simulink model "Constant_TestGen45"  (R2017b)
settings: Solver=FixedStepDiscrete  StartTime=0.0  StopTime=10.0  RelTol=1e-3
settings Model: Creator=ktrinh  LastModifiedBy=ktrinh
settings DebuggingCC: ParameterOverflowMsg=none

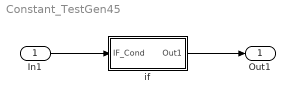
== system Constant_TestGen45 ==
  In1 : Inport
  if : Subsystem  AncestorBlock=Block_TestLib/if
  Out1 : Outport
  wires:
  In1/1 -> if/1(IF_Cond)
  if/1(Out1) -> Out1/1

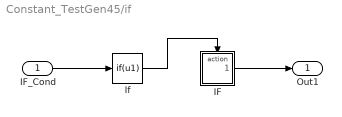
== system Constant_TestGen45/if ==
  IF_Cond : Inport  OutDataTypeStr=boolean
  IF : Subsystem  TreatAsAtomicUnit=on
  If : If  IfExpression=u1  ShowElse=off
  Out1 : Outport
  wires:
  If/1 -> IF/Action
  IF_Cond/1 -> If/1
  IF/1(Out1) -> Out1/1

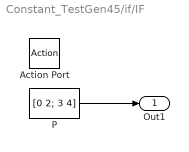
== system Constant_TestGen45/if/IF ==
  Action Port : ActionPort  ActionType=then
  P : Constant  Value=[0 2; 3 4]  VectorParams1D=off  OutDataTypeStr=int32
  Out1 : Outport
  wires:
  P/1 -> Out1/1
